simulink model "E2"  (R2022a)
settings: Solver=VariableStepAuto  StartTime=0.0  StopTime=2*pi  RelTol=1e-3
settings Model: Creator=Reza  LastModifiedBy=Reza

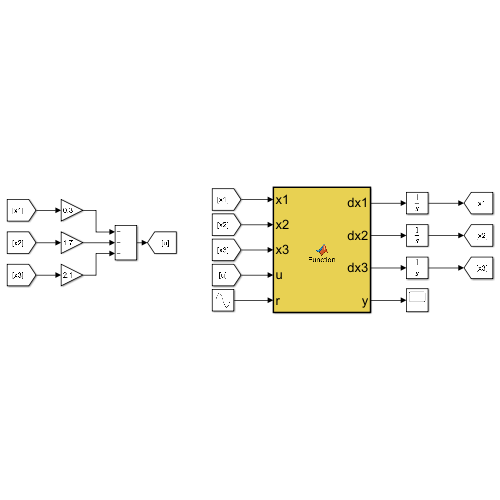
[thumbnail: Simulink's stored preview of the top-level diagram]
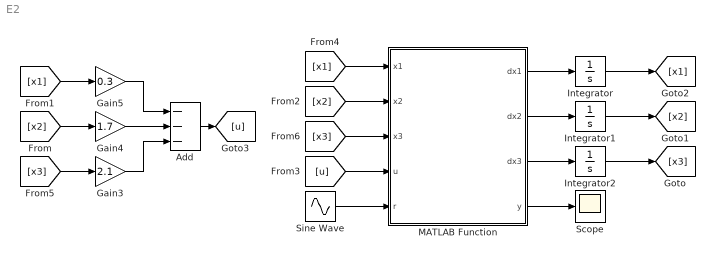
== system E2 ==
  Add : Sum  Inputs=---
  Gain3 : Gain  Gain=2.1
  Gain4 : Gain  Gain=1.7
  Gain5 : Gain  Gain=0.3
  Integrator : Integrator
  Integrator1 : Integrator
  Integrator2 : Integrator
  MATLAB Function : MATLAB Function  TreatAsAtomicUnit=on
  Scope : Scope
  Sine Wave : Sin  SampleTime=0
  wires:
  MATLAB Function/4(y) -> Scope/1
  MATLAB Function/3(dx3) -> Integrator2/1
  MATLAB Function/1(dx1) -> Integrator/1
  MATLAB Function/2(dx2) -> Integrator1/1
  Sine Wave/1 -> MATLAB Function/5(r)
  [x3] -> Gain3/1
  [x2] -> Gain4/1
  [x1] -> Gain5/1
  Integrator2/1 -> [x3]
  Integrator/1 -> [x1]
  Integrator1/1 -> [x2]
  Gain5/1 -> Add/1
  Gain4/1 -> Add/2
  Gain3/1 -> Add/3
  Add/1 -> [u]
  [u] -> MATLAB Function/4(u)
  [x1] -> MATLAB Function/1(x1)
  [x2] -> MATLAB Function/2(x2)
  [x3] -> MATLAB Function/3(x3)

== matlab function E2/MATLAB Function ==
  data: dx1 output; dx2 output; dx3 output; x1 input; y output; x2 input; x3 input; u input; r input
function [dx1,dx2,dx3,y] = Function(x1,x2,x3,u,r)

A = [-2 -1;0 -3];
B = [1;1];
C = [1 3];
a = [A [0;0;];C 0];
b = [B;0];
x = [x1;x2;x3];
dx = a*x+b*u-[0;0;1]*r;
dx1 = dx(1);
dx2 = dx(2);
dx3 = dx(3);
y = x1+3*x2;
